simulink model "Prob_9"  (R2016a)
settings: Solver=VariableStepAuto  StartTime=0.0  StopTime=10.0  RelTol=1e-3
values from neighbouring files (symbols this model uses):
  kt = 0.02    [MAT_file.mat]
undefined symbols (not defined in the file or in its folder): ke
settings Model: Creator=Admin  LastModifiedBy=Admin

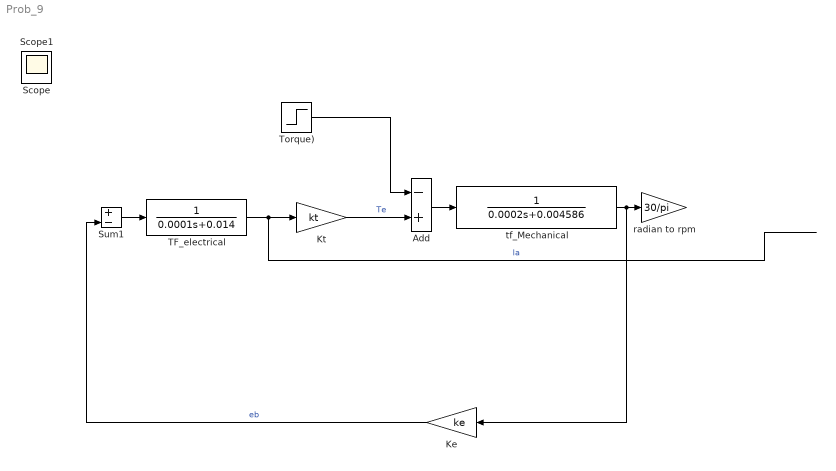
== system Prob_9 ==
  Add : Sum  Inputs=-+
  Ke : Gain  Gain=ke
  Kt : Gain  Gain=kt
  Sum1 : Sum  Inputs=|+-
  "TF_electrical " : TransferFcn  Denominator=[0.0001 0.014]
  Torque) : Step  Time=0.1  After=10  SampleTime=0  ZeroCross=off
  radian to rpm : Gain  Gain=30/pi
  "tf_Mechanical " : TransferFcn  Denominator=[0.0002 0.004586]
  Scope : Scope
  Scope1 : Scope
  wires:
  Sum1/1 -> "TF_electrical "/1
  Kt/1 -> Add/2  "Te"
  Torque)/1 -> Add/1
  Add/1 -> "tf_Mechanical "/1
  "TF_electrical "/1 -> Kt/1  "la"
  Ke/1 -> Sum1/2  "eb"
  "tf_Mechanical "/1 -> Ke/1, radian to rpm/1
